simulink model "lab3_sim"  (R2017a)
settings: Solver=FixedStepAuto  StartTime=0.0  StopTime=2  FixedStep=T  RelTol=1e-3
values from neighbouring files (symbols this model uses):
  A = [0 1 0 0; Amat 0 0 -((Amat*C)/(n*g)); 0 0 0 1; 0 0 0 -C]    [lab3.m]    (also in lab3_ADP.m; lab3_bessel.m)
  B = [0; ((Amat*D)/(n*g)); 0; D]    [lab3.m]    (also in lab3_ADP.m; lab3_bessel.m)
  K = place(phi, gamma, zpoles)    [lab3.m]    (also in lab3_ADP.m; lab3_bessel.m)
  T = 0.01    [lab3.m]    (also in lab3_ADP.m; lab3_bessel.m)
  x1 = [0.17; 0; 0; 0]    [lab3.m]    (also in lab3_ADP.m; lab3_bessel.m)
undefined symbols (not defined in the file or in its folder): Af, Bf, Cf, Df
settings Model: Creator=njohnson  LastModifiedBy=njohnson

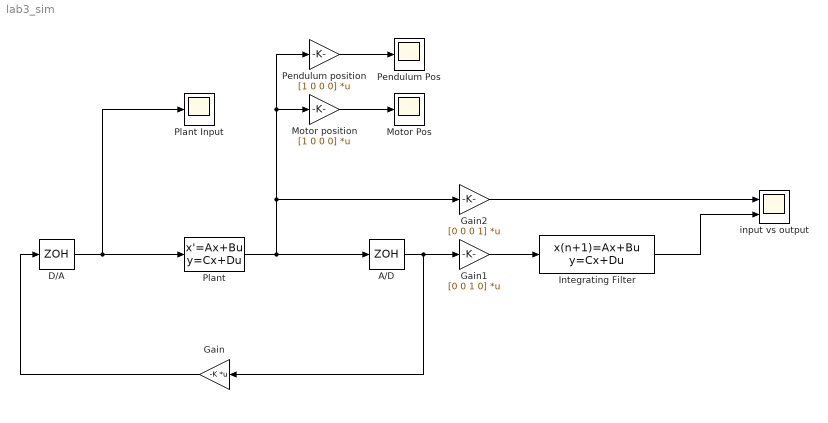
== system lab3_sim ==
  A/D : ZeroOrderHold  SampleTime=T
  D/A : ZeroOrderHold  SampleTime=T
  Gain : Gain  Gain=-K  Multiplication=Matrix(K*u)
  Gain1 : Gain  Gain=[0 0 1 0]  Multiplication=Matrix(K*u)
  Gain2 : Gain  Gain=[0 0 0 1]  Multiplication=Matrix(K*u)
  Integrating Filter : DiscreteStateSpace  A=Af  B=Bf  C=Cf  D=Df  SampleTime=T
  Motor Pos : Scope
  Motor position : Gain  Gain=[1 0 0 0]  Multiplication=Matrix(K*u)
  Pendulum Pos : Scope
  Pendulum position : Gain  Gain=[1 0 0 0]  Multiplication=Matrix(K*u)
  Plant : StateSpace  A=A  B=B  C=eye(4)  D=zeros(4,1)  X0=x1
  "Plant Input " : Scope
  "input vs output " : Scope  NumInputPorts=2
  wires:
  D/A/1 -> "Plant Input "/1, Plant/1
  Plant/1 -> Gain2/1, Pendulum position/1, Motor position/1, A/D/1
  A/D/1 -> Gain1/1, Gain/1
  Gain/1 -> D/A/1
  Pendulum position/1 -> Pendulum Pos/1
  Motor position/1 -> Motor Pos/1
  Gain1/1 -> Integrating Filter/1
  Gain2/1 -> "input vs output "/1
  Integrating Filter/1 -> "input vs output "/2
